simulink model "s299097sim"  (R2022a)
settings: Solver=VariableStepAuto  StartTime=0.0  StopTime=10.0  RelTol=1e-3
libraries: cstblocks x2
settings Model: Creator=S299097  LastModifiedBy=S299097

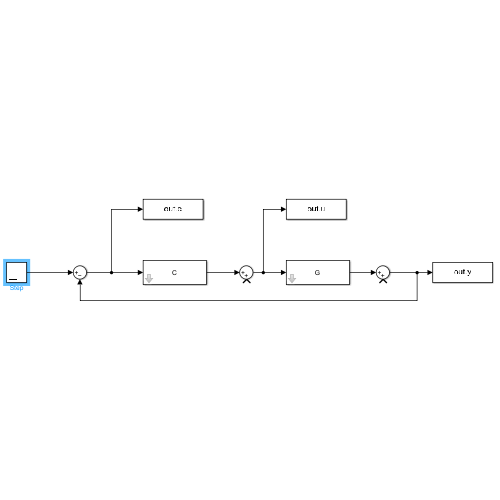
[thumbnail: Simulink's stored preview of the top-level diagram]
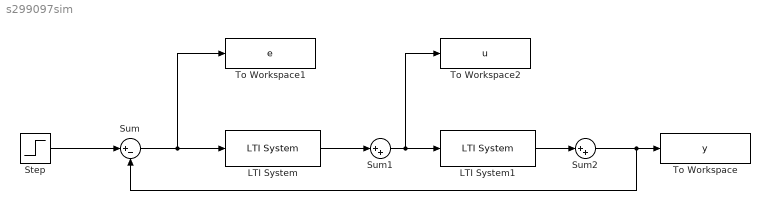
== system s299097sim ==
  LTI System : cstblocks/LTI System  sys=C  IC=[]
  LTI System1 : cstblocks/LTI System  sys=G  IC=[]
  Step : Step  Time=0  SampleTime=0
  Sum : Sum  Inputs=|+-
  Sum1 : Sum  Inputs=|++
  Sum2 : Sum  Inputs=|++
  To Workspace : ToWorkspace  VariableName=y  SaveFormat=Timeseries  SampleTime=-1
  To Workspace1 : ToWorkspace  VariableName=e  SaveFormat=Timeseries  SampleTime=-1
  To Workspace2 : ToWorkspace  VariableName=u  SaveFormat=Timeseries  SampleTime=-1
  wires:
  Step/1 -> Sum/1
  LTI System/1 -> Sum1/1
  Sum1/1 -> To Workspace2/1, LTI System1/1
  Sum/1 -> To Workspace1/1, LTI System/1
  Sum2/1 -> Sum/2, To Workspace/1
  LTI System1/1 -> Sum2/1
